simulink model "trabalhofinal_vR2012a"  (R2012a)
settings: Solver=FixedStepDiscrete  StartTime=0.0  StopTime=0.5  FixedStep=0.1e-6  MaxStep=50e-6
undefined symbols (not defined in the file): DiscIntNeverNeededParam, Ipac0, Vpac0
libraries: powerlib x36, simulink x19, fuzblock x7, powerlib_extras x2, powerlib_meascontrol x2
(part 2 of 3)

== system trabalhofinal_vR2012a/PV array PI/Compensador tensão ==
  Vdc* : Inport
  Vdc : Inport  Port=2
  Bus Creator : BusCreator  Inputs=3
  Constant1 : Constant  Value=Igq_e
  Cv(s) : simulink/Continuous/PID Controller  Controller=PI  TimeDomain=Discrete-time  SampleTime=-1  IntegratorMethod=Trapezoidal  FilterMethod=Forward Euler  Form=Parallel  UseFilter=on  ControllerParametersSource=internal  P=GSC_Cv_kp  I=GSC_Cv_ki  D=0  N=100  InitialConditionSource=external  InitialConditionForIntegrator=0  InitialConditionForFilter=0  ExternalReset=none  LimitOutput=off  UpperSaturationLimit=inf  LowerSaturationLimit=-inf  LinearizeAsGain=on  AntiWindupMode=none  Kb=1  TrackingMode=off  Kt=1  PParamMin=[]  PParamMax=[]  IParamMin=[]  IParamMax=[]  DParamMin=[]  DParamMax=[]  NParamMin=[]  NParamMax=[]  KbParamMin=[]  KbParamMax=[]  KtParamMin=[]  KtParamMax=[]  POutMin=[]  POutMax=[]  IOutMin=[]  IOutMax=[]  DOutMin=[]  DOutMax=[]  NOutMin=[]  NOutMax=[]  KbOutMin=[]  KbOutMax=[]  KtOutMin=[]  KtOutMax=[]  IntegratorOutMin=[]  IntegratorOutMax=[]  FilterOutMin=[]  FilterOutMax=[]  SumOutMin=[]  SumOutMax=[]  SumI1OutMin=[]  SumI1OutMax=[]  SumI2OutMin=[]  SumI2OutMax=[]  SumI3OutMin=[]  SumI3OutMax=[]  SumDOutMin=[]  SumDOutMax=[]  SaturationOutMin=[]  SaturationOutMax=[]  IntegratorContinuousStateAttributes=''  IntegratorStateMustResolveToSignalObject=off  IntegratorRTWStateStorageClass=Auto  FilterContinuousStateAttributes=''  FilterStateMustResolveToSignalObject=off  FilterRTWStateStorageClass=Auto  DifferentiatorICPrevScaledInput=0  DifferentiatorOutMin=[]  DifferentiatorOutMax=[]
  Gain : Gain  Gain=-1
  Scope5 : Scope  NumInputPorts=3
      settings: TimeRange=auto  MaxDataPoints=5000  SaveToWorkspace=off  SaveName=ScopeData2  YMin=2994.84204~2000.00000~589.79398  YMax=3046.42904~4000.00000~1186.78199  SampleTime=-1
  Sum1 : Sum  Inputs=|+-
  igq* : Outport
  DadosCtrlTensao : Outport  Port=2
  wires:
  Constant1/1 -> Cv(s)/2
  Vdc*/1 -> [vdc_ref], Sum1/1  "Vdc*"
  Vdc/1 -> [vdc], Sum1/2  "Vdc"
  Sum1/1 -> Gain/1
  [vdc] -> Scope5/1, Bus Creator/1  "vdc_V"
  [vdc_ref] -> Scope5/2, Bus Creator/2  "vdc_ref_V"
  [iqg_ref] -> Scope5/3, Bus Creator/3  "iqg_ref_A"
  Bus Creator/1 -> DadosCtrlTensao/1
  Gain/1 -> Cv(s)/1
  Cv(s)/1 -> [iqg_ref], igq*/1  "igq*"

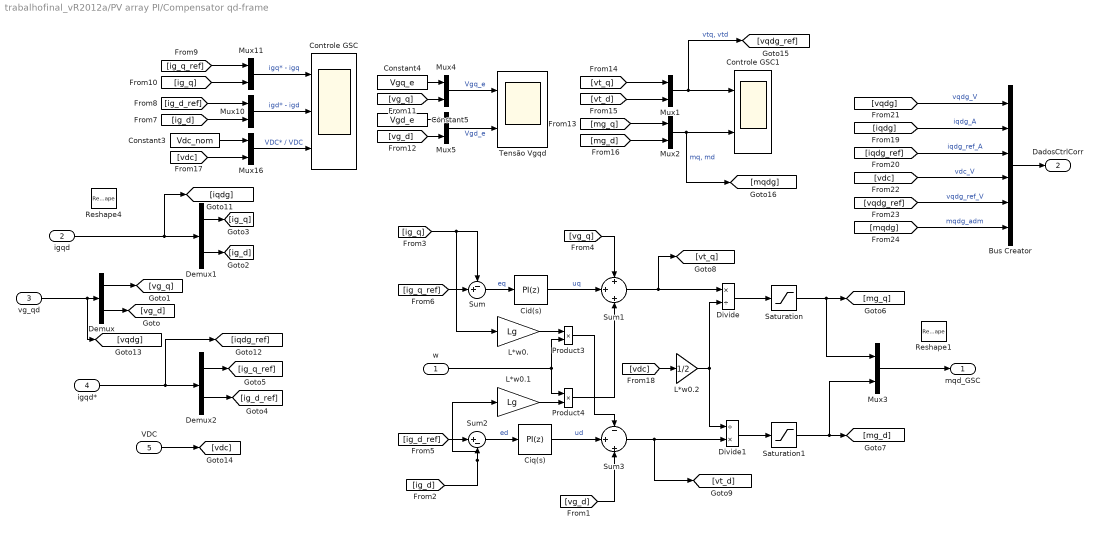
== system trabalhofinal_vR2012a/PV array PI/Compensator qd-frame ==
  w : Inport
  igqd : Inport  Port=2
  vg_qd : Inport  Port=3
  igqd* : Inport  Port=4
  VDC : Inport  Port=5
  Bus Creator : BusCreator  Inputs=6
  Cid(s) : simulink/Continuous/PID Controller  Controller=PI  TimeDomain=Discrete-time  SampleTime=-1  IntegratorMethod=Trapezoidal  FilterMethod=Forward Euler  Form=Parallel  UseFilter=on  ControllerParametersSource=internal  P=GSC_Ci_kp  I=GSC_Ci_ki  D=0  N=100  InitialConditionSource=internal  InitialConditionForIntegrator=GSC_Uq_e  InitialConditionForFilter=0  ExternalReset=none  LimitOutput=off  UpperSaturationLimit=inf  LowerSaturationLimit=-inf  LinearizeAsGain=on  AntiWindupMode=none  Kb=1  TrackingMode=off  Kt=1  PParamMin=[]  PParamMax=[]  IParamMin=[]  IParamMax=[]  DParamMin=[]  DParamMax=[]  NParamMin=[]  NParamMax=[]  KbParamMin=[]  KbParamMax=[]  KtParamMin=[]  KtParamMax=[]  POutMin=[]  POutMax=[]  IOutMin=[]  IOutMax=[]  DOutMin=[]  DOutMax=[]  NOutMin=[]  NOutMax=[]  KbOutMin=[]  KbOutMax=[]  KtOutMin=[]  KtOutMax=[]  IntegratorOutMin=[]  IntegratorOutMax=[]  FilterOutMin=[]  FilterOutMax=[]  SumOutMin=[]  SumOutMax=[]  SumI1OutMin=[]  SumI1OutMax=[]  SumI2OutMin=[]  SumI2OutMax=[]  SumI3OutMin=[]  SumI3OutMax=[]  SumDOutMin=[]  SumDOutMax=[]  SaturationOutMin=[]  SaturationOutMax=[]  IntegratorContinuousStateAttributes=''  IntegratorStateMustResolveToSignalObject=off  IntegratorRTWStateStorageClass=Auto  FilterContinuousStateAttributes=''  FilterStateMustResolveToSignalObject=off  FilterRTWStateStorageClass=Auto  DifferentiatorICPrevScaledInput=0  DifferentiatorOutMin=[]  DifferentiatorOutMax=[]
  Ciq(s) : simulink/Continuous/PID Controller  Controller=PI  TimeDomain=Discrete-time  SampleTime=-1  IntegratorMethod=Trapezoidal  FilterMethod=Forward Euler  Form=Parallel  UseFilter=on  ControllerParametersSource=internal  P=GSC_Ci_kp  I=GSC_Ci_ki  D=0  N=100  InitialConditionSource=internal  InitialConditionForIntegrator=GSC_Ud_e  InitialConditionForFilter=0  ExternalReset=none  LimitOutput=off  UpperSaturationLimit=inf  LowerSaturationLimit=-inf  LinearizeAsGain=on  AntiWindupMode=none  Kb=1  TrackingMode=off  Kt=1  PParamMin=[]  PParamMax=[]  IParamMin=[]  IParamMax=[]  DParamMin=[]  DParamMax=[]  NParamMin=[]  NParamMax=[]  KbParamMin=[]  KbParamMax=[]  KtParamMin=[]  KtParamMax=[]  POutMin=[]  POutMax=[]  IOutMin=[]  IOutMax=[]  DOutMin=[]  DOutMax=[]  NOutMin=[]  NOutMax=[]  KbOutMin=[]  KbOutMax=[]  KtOutMin=[]  KtOutMax=[]  IntegratorOutMin=[]  IntegratorOutMax=[]  FilterOutMin=[]  FilterOutMax=[]  SumOutMin=[]  SumOutMax=[]  SumI1OutMin=[]  SumI1OutMax=[]  SumI2OutMin=[]  SumI2OutMax=[]  SumI3OutMin=[]  SumI3OutMax=[]  SumDOutMin=[]  SumDOutMax=[]  SaturationOutMin=[]  SaturationOutMax=[]  IntegratorContinuousStateAttributes=''  IntegratorStateMustResolveToSignalObject=off  IntegratorRTWStateStorageClass=Auto  FilterContinuousStateAttributes=''  FilterStateMustResolveToSignalObject=off  FilterRTWStateStorageClass=Auto  DifferentiatorICPrevScaledInput=0  DifferentiatorOutMin=[]  DifferentiatorOutMax=[]
  Constant3 : Constant  Value=Vdc_nom
  Constant4 : Constant  Value=Vgq_e
  Constant5 : Constant  Value=Vgd_e
  Controle GSC : Scope  NumInputPorts=3
      settings: TimeRange=0.1  MaxDataPoints=5000  SaveToWorkspace=off  SaveName=ScopeData3  YMin=-63.17117~-5.51729~796.71882  YMax=425.59411~20.68997~829.53063  SampleTime=-1
  Controle GSC1 : Scope  NumInputPorts=2
      settings: TimeRange=auto  MaxDataPoints=5000  SaveToWorkspace=off  SaveName=ScopeData4  YMin=-135.91868~-0.45232  YMax=350.40738~1.16137  SampleTime=-1
  Demux : Demux  Outputs=2
  Demux1 : Demux  Outputs=2
  Demux2 : Demux  Outputs=2
  Divide : Product  Inputs=*/
  Divide1 : Product  Inputs=/*
  L*w0. : Gain  Gain=Lg
  L*w0.1 : Gain  Gain=Lg
  L*w0.2 : Gain  Gain=1/2
  Mux{1..5,10..11,16} (8 alike) : Mux  Inputs=2
  Product3 : Product
  Product4 : Product
  Reshape1 : Reshape  OutputDimensionality=Customize  OutputDimensions=[2,1]
  Reshape4 : Reshape  OutputDimensionality=Customize  OutputDimensions=[2,1]
  Saturation : Saturate  UpperLimit=1  LowerLimit=-1
  Saturation1 : Saturate  UpperLimit=1  LowerLimit=-1
  Sum : Sum  Inputs=-+|
  Sum1 : Sum  Inputs=+|+|+
  Sum2 : Sum  Inputs=|+-
  Sum3 : Sum  Inputs=-|+|+
  Tensão Vgqd : Scope  NumInputPorts=2
      settings: TimeRange=auto  MaxDataPoints=5000  SaveToWorkspace=off  SaveName=ScopeData36  YMin=148.66619~-14.34464  YMax=209.64626~12.14165  SampleTime=-1
  mqd_GSC : Outport
  DadosCtrlCorr : Outport  Port=2
  wires:
  Demux/2 -> [vg_d]
  Demux/1 -> [vg_q]
  Demux1/2 -> [ig_d]
  Demux1/1 -> [ig_q]
  L*w0.2/1 -> Divide/2, Divide1/1
  [mg_q] -> Mux2/1
  [mg_d] -> Mux2/2
  [vt_q] -> Mux1/1
  [vt_d] -> Mux1/2
  Mux2/1 -> [mqdg], Controle GSC1/2  "mq, md"
  Mux1/1 -> [vqdg_ref], Controle GSC1/1  "vtq, vtd"
  [ig_q] -> Mux11/2
  [ig_q_ref] -> Mux11/1
  [ig_d] -> Mux10/2
  [ig_d_ref] -> Mux10/1
  Mux11/1 -> Controle GSC/1  "igq* - igq"
  Mux10/1 -> Controle GSC/2  "igd* - igd"
  Divide/1 -> Saturation/1
  L*w0.1/1 -> Product4/2
  [ig_q_ref] -> Sum/2
  igqd*/1 -> Demux2/1, [iqdg_ref]
  VDC/1 -> [vdc]
  Sum/1 -> Cid(s)/1  "eq"
  [ig_d] -> L*w0.1/1, Sum2/2
  Sum1/1 -> Divide/1, [vt_q]
  Cid(s)/1 -> Sum1/2  "uq"
  Ciq(s)/1 -> Sum3/2  "ud"
  Sum2/1 -> Ciq(s)/1  "ed"
  Sum3/1 -> Divide1/2, [vt_d]
  L*w0./1 -> Product3/1
  [ig_d_ref] -> Sum2/1
  Mux16/1 -> Controle GSC/3  "VDC* / VDC"
  Constant3/1 -> Mux16/1
  [vdc] -> Mux16/2
  Demux2/1 -> [ig_q_ref]
  Demux2/2 -> [ig_d_ref]
  [vdc] -> L*w0.2/1
  Constant4/1 -> Mux4/1
  [vg_q] -> Mux4/2
  Constant5/1 -> Mux5/1
  [vg_d] -> Mux5/2
  Mux4/1 -> Tensão Vgqd/1  "Vgq_e"
  Mux5/1 -> Tensão Vgqd/2  "Vgd_e"
  Saturation/1 -> Mux3/1, [mg_q]
  Divide1/1 -> Saturation1/1
  Saturation1/1 -> Mux3/2, [mg_d]
  [ig_q] -> Sum/1, L*w0./1
  igqd/1 -> [iqdg], Demux1/1
  vg_qd/1 -> [vqdg], Demux/1
  Mux3/1 -> mqd_GSC/1
  [vqdg] -> Bus Creator/1  "vqdg_V"
  [iqdg] -> Bus Creator/2  "iqdg_A"
  [iqdg_ref] -> Bus Creator/3  "iqdg_ref_A"
  Bus Creator/1 -> DadosCtrlCorr/1
  [vdc] -> Bus Creator/4  "vdc_V"
  [vqdg_ref] -> Bus Creator/5  "vqdg_ref_V"
  [mqdg] -> Bus Creator/6  "mqdg_adm"
  [vg_q] -> Sum1/1
  [vg_d] -> Sum3/3
  Product3/1 -> Sum3/1
  Product4/1 -> Sum1/3
  w/1 -> Product3/2, Product4/1

== system trabalhofinal_vR2012a/PV array PI/DSOGI1 ==
  note: Fasor = (Fq-jFd)/sqrt(2)
  angV : Inport
  V : Inport  Port=2
  I : Inport  Port=3
  Calcula Impedância2 : Subsystem
  Complex to Magnitude-Angle : ComplexToMagnitudeAngle  Output=Angle
  Complex to Magnitude-Angle1 : ComplexToMagnitudeAngle
  Fasor_Krause : Subsystem
  Fasor_Krause1 : Subsystem
  Magnitude-Angle to Complex : MagnitudeAngleToComplex
  Sum : Sum  Inputs=|++
  Terminator : Terminator
  I_fasor : Outport
  wires:
  Magnitude-Angle to Complex/1 -> I_fasor/1
  Complex to Magnitude-Angle1/2 -> Sum/1
  Complex to Magnitude-Angle1/1 -> Magnitude-Angle to Complex/1
  Complex to Magnitude-Angle/1 -> Terminator/1
  V/1 -> Calcula Impedância2/1(Vinf_abc)
  I/1 -> Calcula Impedância2/2(I_abc)
  Calcula Impedância2/1(Vinf_q) -> Fasor_Krause/1(Fq)
  Calcula Impedância2/2(Vinf_d) -> Fasor_Krause/2(Fd)
  Fasor_Krause/1(Fasor) -> Complex to Magnitude-Angle/1
  Calcula Impedância2/3(Ipac_q) -> Fasor_Krause1/1(Fq)
  Calcula Impedância2/4(Ipac_d) -> Fasor_Krause1/2(Fd)
  Fasor_Krause1/1(Fasor) -> Complex to Magnitude-Angle1/1
  Sum/1 -> Magnitude-Angle to Complex/2
  angV/1 -> Sum/2

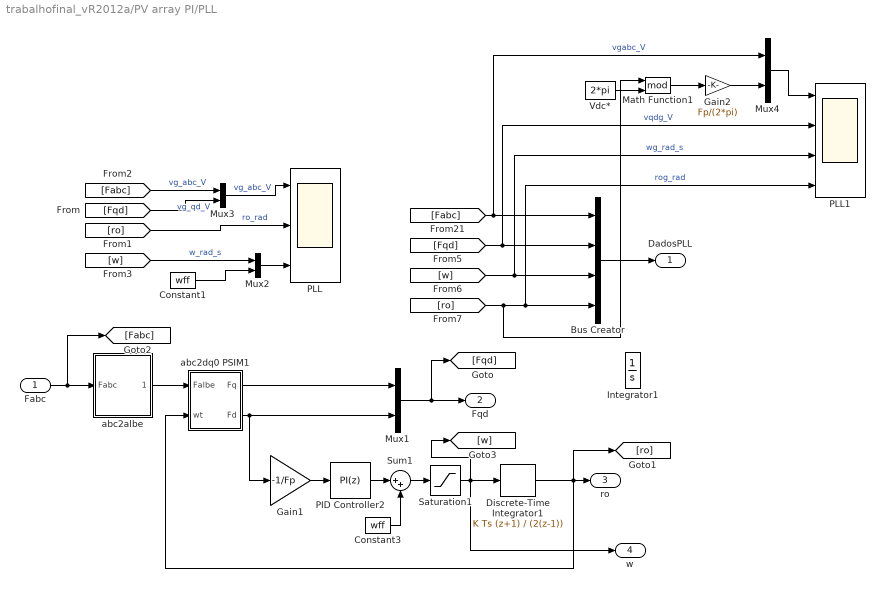
== system trabalhofinal_vR2012a/PV array PI/PLL ==
  Fabc : Inport
  Bus Creator : BusCreator  Inputs=4
  Constant1 : Constant  Value=wff
  Constant3 : Constant  Value=wff
  Discrete-Time Integrator1 : DiscreteIntegrator  IntegratorMethod=Integration: Trapezoidal  InitialCondition=ro0  InitialConditionMode=State only (most efficient)  SampleTime=-1  ICPrevOutput=DiscIntNeverNeededParam  ICPrevScaledInput=DiscIntNeverNeededParam
  Gain1 : Gain  Gain=-1/Fp
  Gain2 : Gain  Gain=Fp/(2*pi)
  Integrator1 : Integrator  InitialCondition=ro0  UpperSaturationLimit=2*pi  LowerSaturationLimit=0
  Math Function1 : Math  Operator=mod  SaturateOnIntegerOverflow=on
  Mux{1..4} (4 alike) : Mux  Inputs=2
  PID Controller2 : simulink/Continuous/PID Controller  Controller=PI  TimeDomain=Discrete-time  SampleTime=-1  IntegratorMethod=Trapezoidal  FilterMethod=Forward Euler  Form=Parallel  UseFilter=on  ControllerParametersSource=internal  P=kp  I=ki  D=1  N=100  InitialConditionSource=internal  InitialConditionForIntegrator=dw0  InitialConditionForFilter=0  ExternalReset=none  LimitOutput=off  UpperSaturationLimit=inf  LowerSaturationLimit=-inf  LinearizeAsGain=on  AntiWindupMode=none  Kb=1  TrackingMode=off  Kt=1  PParamMin=[]  PParamMax=[]  IParamMin=[]  IParamMax=[]  DParamMin=[]  DParamMax=[]  NParamMin=[]  NParamMax=[]  KbParamMin=[]  KbParamMax=[]  KtParamMin=[]  KtParamMax=[]  POutMin=[]  POutMax=[]  IOutMin=[]  IOutMax=[]  DOutMin=[]  DOutMax=[]  NOutMin=[]  NOutMax=[]  KbOutMin=[]  KbOutMax=[]  KtOutMin=[]  KtOutMax=[]  IntegratorOutMin=[]  IntegratorOutMax=[]  FilterOutMin=[]  FilterOutMax=[]  SumOutMin=[]  SumOutMax=[]  SumI1OutMin=[]  SumI1OutMax=[]  SumI2OutMin=[]  SumI2OutMax=[]  SumI3OutMin=[]  SumI3OutMax=[]  SumDOutMin=[]  SumDOutMax=[]  SaturationOutMin=[]  SaturationOutMax=[]  IntegratorContinuousStateAttributes=''  IntegratorStateMustResolveToSignalObject=off  IntegratorRTWStateStorageClass=Auto  FilterContinuousStateAttributes=''  FilterStateMustResolveToSignalObject=off  FilterRTWStateStorageClass=Auto  DifferentiatorICPrevScaledInput=0  DifferentiatorOutMin=[]  DifferentiatorOutMax=[]
  PLL : Scope  NumInputPorts=3
      settings: TimeRange=auto  MaxDataPoints=5000  SaveToWorkspace=off  SaveName=ScopeData  YMin=-224.53656~-6.47953~126.78086  YMax=224.53656~42.60785~2394.62118  SampleTime=-1
  PLL1 : Scope  NumInputPorts=4
      settings: TimeRange=auto  MaxDataPoints=5000  SaveToWorkspace=off  SaveName=ScopeData2  YMin=-449.07312~-45.53757~341.99428~-25.11328  YMax=449.07312~404.23584~381.19293~210.48455  SampleTime=-1
  Saturation1 : Saturate  UpperLimit=10*wff  LowerLimit=-0.1*wff
  Sum1 : Sum  Inputs=|++
  Vdc* : Constant  Value=2*pi  SampleTime=-1
  abc2albe : Subsystem
  abc2dq0 PSIM1 : Subsystem
  DadosPLL : Outport
  Fqd : Outport  Port=2
  ro : Outport  Port=3
  w : Outport  Port=4
  wires:
  abc2albe/1(Falbe) -> abc2dq0 PSIM1/1(Falbe)
  abc2dq0 PSIM1/2(Fd) -> Gain1/1, Mux1/2
  Constant3/1 -> Sum1/2
  abc2dq0 PSIM1/1(Fq) -> Mux1/1
  Sum1/1 -> Saturation1/1
  Gain1/1 -> PID Controller2/1
  PID Controller2/1 -> Sum1/1
  Mux3/1 -> PLL/1  "vg_abc_V"
  Fabc/1 -> abc2albe/1(Fabc), [Fabc]
  [ro] -> PLL/2  "ro_rad"
  [Fqd] -> Mux3/2  "vg_qd_V"
  Mux1/1 -> Fqd/1, [Fqd]
  [w] -> Mux2/1  "w_rad_s"
  Mux2/1 -> PLL/3
  Constant1/1 -> Mux2/2
  [Fabc] -> Mux4/1, Bus Creator/1  "vgabc_V"
  [Fqd] -> PLL1/2, Bus Creator/2  "vqdg_V"
  [w] -> PLL1/3, Bus Creator/3  "wg_rad_s"
  Bus Creator/1 -> DadosPLL/1
  [ro] -> Math Function1/1, PLL1/4, Bus Creator/4  "rog_rad"
  [Fabc] -> Mux3/1  "vg_abc_V"
  Saturation1/1 -> w/1, Discrete-Time Integrator1/1, [w]
  Discrete-Time Integrator1/1 -> [ro], abc2dq0 PSIM1/2(wt), ro/1
  Vdc*/1 -> Math Function1/2
  Math Function1/1 -> Gain2/1
  Mux4/1 -> PLL1/1
  Gain2/1 -> Mux4/2

== system trabalhofinal_vR2012a/PV array PI/PWM ==
  mabc : Inport
  PWM Generator1 : powerlib_extras/Control  Blocks/PWM Generator  GeneratorMode="3-arm  bridge (6 pulses)"  Fc=PWM_freq_grid  Internal=off  mIndex=0.4  Freq=60  Phase=0
  Unit Delay4 : UnitDelay  SampleTime=-1
  Pulses : Outport
  wires:
  PWM Generator1/1 -> Pulses/1
  mabc/1 -> PWM Generator1/1

== system trabalhofinal_vR2012a/PV array PI/Subsystem ==
  Current Measurement : powerlib/Measurements/Current Measurement  PhasorSimulation=off  OutputType=Complex  PSBequivalent=0
  vbn : powerlib/Measurements/Voltage Measurement  PhasorSimulation=off  OutputType=Complex  PSBequivalent=0
  A : PMIOPort  Port=1  Side=Left
  a : PMIOPort  Port=2  Side=Right
  B : PMIOPort  Port=3  Side=Left
  Vdc : Outport
  Idc : Outport  Port=2
  wires:
  Current Measurement/1 -> Idc/1
  vbn/1 -> Vdc/1
  connections:
  Current Measurement/LConn1 -- a/RConn1
  vbn/LConn2 -- B/RConn1
  vbn/LConn1 -- A/RConn1 -- Current Measurement/RConn1

== system trabalhofinal_vR2012a/PV array PI/abc2dq0 PSIM1 ==
  Fabc : Inport
  wt : Inport  Port=2
  Mux1 : Mux  Inputs=2
  abc2albe : Subsystem
  abc2dq0 PSIM1 : Subsystem
  Fqd : Outport
  wires:
  abc2albe/1(Falbe) -> abc2dq0 PSIM1/1(Falbe)
  abc2dq0 PSIM1/2(Fd) -> Mux1/2
  abc2dq0 PSIM1/1(Fq) -> Mux1/1
  Mux1/1 -> Fqd/1
  wt/1 -> abc2dq0 PSIM1/2(wt)
  Fabc/1 -> abc2albe/1(Fabc)

== system trabalhofinal_vR2012a/PV array PI/dq02abc PSIM ==
  Fqd : Inport
  wt : Inport  Port=2
  abc2dq0 PSIM : Subsystem
  albe2abc : Subsystem
  Fabc : Outport
  wires:
  albe2abc/1(Fabc) -> Fabc/1
  abc2dq0 PSIM/1(Falbe) -> albe2abc/1(Falbe)
  wt/1 -> abc2dq0 PSIM/2(wt)
  Fqd/1 -> abc2dq0 PSIM/1(Fqd)

== system trabalhofinal_vR2012a/PV array Fuzzy/Compensador tensão/F1 ==
  E : Inport
  Fuzzy Logic Controller1 : fuzblock/Fuzzy Logic  Controller  fis=fuzzyControl
  Gain9 : Gain  Gain=GY
  Mux6 : Mux  Inputs=2
  Rate Transition1 : RateTransition  OutPortSampleTime=Ts_fuzzy
  Rate Transition2 : RateTransition
  Saturation2 : Saturate  UpperLimit=1  LowerLimit=-1
  Scope5 : Scope  NumInputPorts=3
      settings: TimeRange=auto  MaxDataPoints=5000  SaveToWorkspace=off  YMin=-1.25~-0.09079~-1.05  YMax=1.25~0.07544~1.05  SampleTime=-1
  Subsystem1 : Subsystem
  u : Outport
  wires:
  Rate Transition1/1 -> Subsystem1/1(E)
  Saturation2/1 -> Gain9/1
  Subsystem1/1(E.) -> Mux6/1, Scope5/1  "E"
  Mux6/1 -> Fuzzy Logic Controller1/1
  Subsystem1/2(CE) -> Mux6/2, Scope5/2  "CE"
  Fuzzy Logic Controller1/1 -> Scope5/3, Saturation2/1  "u"
  Gain9/1 -> Rate Transition2/1
  E/1 -> Rate Transition1/1
  Rate Transition2/1 -> u/1

== system trabalhofinal_vR2012a/PV array Fuzzy/Compensador tensão/F2 ==
  E : Inport
  Fuzzy Logic Controller1 : fuzblock/Fuzzy Logic  Controller  fis=fuzzyControl
  Gain9 : Gain  Gain=GY
  Mux6 : Mux  Inputs=2
  Rate Transition1 : RateTransition  OutPortSampleTime=Ts_fuzzy
  Rate Transition2 : RateTransition
  Saturation2 : Saturate  UpperLimit=1  LowerLimit=-1
  Scope5 : Scope  NumInputPorts=3
      settings: TimeRange=auto  MaxDataPoints=5000  SaveToWorkspace=off  YMin=-1.25~-0.66794~-1.05  YMax=1.25~1.18533~1.05  SampleTime=-1
  Subsystem1 : Subsystem
  u : Outport
  wires:
  Rate Transition2/1 -> u/1
  E/1 -> Rate Transition1/1
  Gain9/1 -> Rate Transition2/1
  Fuzzy Logic Controller1/1 -> Saturation2/1, Scope5/3  "u"
  Subsystem1/2(CE) -> Scope5/2, Mux6/2  "CE"
  Mux6/1 -> Fuzzy Logic Controller1/1
  Subsystem1/1(E.) -> Scope5/1, Mux6/1  "E"
  Saturation2/1 -> Gain9/1
  Rate Transition1/1 -> Subsystem1/1(E)

== system trabalhofinal_vR2012a/PV array Fuzzy/Compensador tensão/F3 ==
  E : Inport
  Fuzzy Logic Controller1 : fuzblock/Fuzzy Logic  Controller  fis=fuzzyControl
  Gain9 : Gain  Gain=GY
  Mux6 : Mux  Inputs=2
  Rate Transition1 : RateTransition  OutPortSampleTime=Ts_fuzzy
  Rate Transition2 : RateTransition
  Saturation2 : Saturate  UpperLimit=1  LowerLimit=-1
  Scope5 : Scope  NumInputPorts=3
      settings: TimeRange=auto  MaxDataPoints=5000  SaveToWorkspace=off  YMin=-0.08604~-0.00307~-0.07636  YMax=0.77447~0.01457~0.68814  SampleTime=-1
  Subsystem1 : Subsystem
  u : Outport
  wires:
  Rate Transition1/1 -> Subsystem1/1(E)
  Saturation2/1 -> Gain9/1
  Subsystem1/1(E.) -> Mux6/1, Scope5/1  "E"
  Mux6/1 -> Fuzzy Logic Controller1/1
  Subsystem1/2(CE) -> Mux6/2, Scope5/2  "CE"
  Fuzzy Logic Controller1/1 -> Scope5/3, Saturation2/1  "u"
  Gain9/1 -> Rate Transition2/1
  E/1 -> Rate Transition1/1
  Rate Transition2/1 -> u/1

== system trabalhofinal_vR2012a/PV array Fuzzy/Compensador tensão/F4 ==
  E : Inport
  Fuzzy Logic Controller1 : fuzblock/Fuzzy Logic  Controller  fis=fuzzyControl
  Gain9 : Gain  Gain=GY
  Mux6 : Mux  Inputs=2
  Rate Transition1 : RateTransition  OutPortSampleTime=Ts_fuzzy
  Rate Transition2 : RateTransition
  Saturation2 : Saturate  UpperLimit=1  LowerLimit=-1
  Scope5 : Scope  NumInputPorts=3
      settings: TimeRange=auto  MaxDataPoints=5000  SaveToWorkspace=off  YMin=-0.0901~-0.00492~-0.07806  YMax=0.81164~0.01477~0.70508  SampleTime=-1
  Subsystem1 : Subsystem
  u : Outport
  wires:
  Rate Transition1/1 -> Subsystem1/1(E)
  Saturation2/1 -> Gain9/1
  Subsystem1/1(E.) -> Mux6/1, Scope5/1  "E"
  Mux6/1 -> Fuzzy Logic Controller1/1
  Subsystem1/2(CE) -> Mux6/2, Scope5/2  "CE"
  Fuzzy Logic Controller1/1 -> Scope5/3, Saturation2/1  "u"
  Gain9/1 -> Rate Transition2/1
  E/1 -> Rate Transition1/1
  Rate Transition2/1 -> u/1

== system trabalhofinal_vR2012a/PV array Fuzzy/Compensador tensão/Ganhos1 ==
  E : Inport
  Fuzzy Logic Controller1 : fuzblock/Fuzzy Logic  Controller  fis=fuzzyControl
  Gain9 : Gain  Gain=GY
  Mux6 : Mux  Inputs=2
  Rate Transition1 : RateTransition  OutPortSampleTime=Ts_fuzzy
  Saturation2 : Saturate  UpperLimit=1  LowerLimit=-1
  Scope5 : Scope  NumInputPorts=3
      settings: TimeRange=auto  MaxDataPoints=5000  SaveToWorkspace=off  YMin=-0.36602~-1.25~-1.04912  YMax=0.83247~1.25~1.04987  SampleTime=-1
  Subsystem1 : Subsystem
  u : Outport
  wires:
  Gain9/1 -> u/1
  E/1 -> Rate Transition1/1
  Fuzzy Logic Controller1/1 -> Saturation2/1, Scope5/3  "u"
  Subsystem1/2(CE) -> Scope5/2, Mux6/2  "CE"
  Mux6/1 -> Fuzzy Logic Controller1/1
  Subsystem1/1(E.) -> Scope5/1, Mux6/1  "E"
  Saturation2/1 -> Gain9/1
  Rate Transition1/1 -> Subsystem1/1(E)

== system trabalhofinal_vR2012a/PV array Fuzzy/Compensador tensão/Subsystem1 ==
  E : Inport
  Discrete Derivative1 : simulink/Discrete/Discrete Derivative  gainval=1  ICPrevScaledInput=0.0  OutMin=[]  OutMax=[]  OutDataType=fixdt(1, 16)  OutScaling=2^-10  DoSatur=off
  E. : Outport
  CE : Outport  Port=2
  wires:
  E/1 -> E./1, Discrete Derivative1/1
  Discrete Derivative1/1 -> CE/1  "CE"

== system trabalhofinal_vR2012a/PV array Fuzzy/Compensador tensão/razoável ==
  E : Inport
  Fuzzy Logic Controller1 : fuzblock/Fuzzy Logic  Controller  fis=teste03
  Gain9 : Gain  Gain=GY
  Mux6 : Mux  Inputs=2
  Rate Transition1 : RateTransition  OutPortSampleTime=0.0001
  Rate Transition2 : RateTransition
  Saturation2 : Saturate  UpperLimit=1  LowerLimit=-1
  Scope5 : Scope  NumInputPorts=3
      settings: TimeRange=auto  MaxDataPoints=5000  SaveToWorkspace=off  YMin=-0.03774~-0.02191~-0.05244  YMax=0.33999~0.07353~0.47629  SampleTime=-1
  Subsystem1 : Subsystem
  u : Outport
  wires:
  Saturation2/1 -> Gain9/1
  Subsystem1/1(E.) -> Mux6/1, Scope5/1  "E"
  Mux6/1 -> Fuzzy Logic Controller1/1
  Subsystem1/2(CE) -> Mux6/2, Scope5/2  "CE"
  Fuzzy Logic Controller1/1 -> Scope5/3, Saturation2/1  "u"
  Gain9/1 -> Rate Transition2/1
  E/1 -> Rate Transition1/1
  Rate Transition1/1 -> Subsystem1/1(E)
  Rate Transition2/1 -> u/1

== system trabalhofinal_vR2012a/PV array Fuzzy/Compensator qd-frame/FuzzyControl_q3 ==
  E : Inport
  Fuzzy Logic Controller1 : fuzblock/Fuzzy Logic  Controller  fis=teste03
  Gain9 : Gain  Gain=GY
  Mux6 : Mux  Inputs=2
  Rate Transition1 : RateTransition  OutPortSampleTime=0.0001
  Rate Transition2 : RateTransition
  Saturation2 : Saturate  UpperLimit=1  LowerLimit=-1
  Scope5 : Scope  NumInputPorts=3
      settings: TimeRange=auto  MaxDataPoints=5000  SaveToWorkspace=off  YMin=-0.34895~-1.25~-1.04994  YMax=1.14988~1.25~1.04999  SampleTime=-1
  Subsystem1 : Subsystem
  u : Outport
  wires:
  Rate Transition2/1 -> u/1
  Rate Transition1/1 -> Subsystem1/1(E)
  E/1 -> Rate Transition1/1
  Gain9/1 -> Rate Transition2/1
  Fuzzy Logic Controller1/1 -> Saturation2/1, Scope5/3  "u"
  Subsystem1/2(CE) -> Scope5/2, Mux6/2  "CE"
  Mux6/1 -> Fuzzy Logic Controller1/1
  Subsystem1/1(E.) -> Scope5/1, Mux6/1  "E"
  Saturation2/1 -> Gain9/1

== system trabalhofinal_vR2012a/PV array Fuzzy/Compensator qd-frame/Subsystem2 ==
  E : Inport
  Discrete Derivative1 : simulink/Discrete/Discrete Derivative  gainval=1  ICPrevScaledInput=0.0  OutMin=[]  OutMax=[]  OutDataType=fixdt(1, 16)  OutScaling=2^-10  DoSatur=off
  Gain8 : Gain
  Gain9 : Gain
  Saturation2 : Saturate  UpperLimit=inf  LowerLimit=-inf
  E. : Outport
  CE : Outport  Port=2
  wires:
  Gain9/1 -> E./1
  Saturation2/1 -> CE/1
  E/1 -> Discrete Derivative1/1, Gain9/1
  Discrete Derivative1/1 -> Gain8/1  "CE"
  Gain8/1 -> Saturation2/1

== system trabalhofinal_vR2012a/PV array Fuzzy/DSOGI1/Calcula Impedância2 ==
  Vinf_abc : Inport
  I_abc : Inport  Port=2
  Constant2 : Constant  Value=wB  SampleTime=0
  DSOGI (Corrente) : Subsystem
  DSOGI (Tensão) : Subsystem
  Demux : Demux  Outputs=2
  Demux1 : Demux  Outputs=2
  Gain : Gain
  PLL : Subsystem
  PLL1 : Scope  NumInputPorts=2
      settings: TimeRange=auto  MaxDataPoints=5000  SaveToWorkspace=off  SaveName=ScopeData5  YMin=-1.5~-0.25  YMax=1.5~1.5  SampleTime=-1
  PLL2 : Scope  NumInputPorts=2
      settings: TimeRange=auto  MaxDataPoints=5000  SaveToWorkspace=off  YMin=-1.5~-0.25  YMax=1.5~1.5  SampleTime=-1
  Sum1 : Sum  Inputs=+-|
  Terminator6 : Terminator
  Terminator7 : Terminator
  abc2albe : Subsystem
  abc2albe1 : Subsystem
  abc2dq0 PSIM : Subsystem
  Vinf_q : Outport
  Vinf_d : Outport  Port=2
  Ipac_q : Outport  Port=3
  Ipac_d : Outport  Port=4
  wires:
  Gain/1 -> Sum1/2
  I_abc/1 -> abc2albe1/1(Fabc)
  PLL/3(ro) -> PLL/2(wt), abc2dq0 PSIM/2(wt)
  DSOGI (Corrente)/1(Falbe(+)) -> PLL1/1, abc2dq0 PSIM/1(Falbe)
  DSOGI (Corrente)/2(Falbe(-)) -> Terminator7/1
  abc2albe1/1(Falbe) -> DSOGI (Corrente)/2(Falbe)
  DSOGI (Tensão)/2(Falbe(-)) -> Terminator6/1
  Vinf_abc/1 -> abc2albe/1(Fabc)
  DSOGI (Tensão)/1(Falbe(+)) -> PLL/1(Falbe)
  abc2albe/1(Falbe) -> DSOGI (Tensão)/2(Falbe)
  PLL/1(Fqd) -> Demux/1, PLL2/1
  Demux1/2 -> Ipac_d/1
  Demux/2 -> Vinf_d/1
  Demux/1 -> Vinf_q/1
  abc2dq0 PSIM/1(Fqd) -> PLL1/2, Demux1/1
  Demux1/1 -> Ipac_q/1
  PLL/2(w) -> PLL2/2
  Constant2/1 -> DSOGI (Corrente)/1(w), DSOGI (Tensão)/1(w)

== system trabalhofinal_vR2012a/PV array Fuzzy/DSOGI1/Fasor_Krause ==
  Fq : Inport
  Fd : Inport  Port=2
  Gain12 : Gain  Gain=-1
  Gain7 : Gain  Gain=1/sqrt(2)
  Real-Imag to Complex1 : RealImagToComplex
  Fasor : Outport
  wires:
  Real-Imag to Complex1/1 -> Gain7/1
  Fq/1 -> Real-Imag to Complex1/1
  Gain12/1 -> Real-Imag to Complex1/2
  Fd/1 -> Gain12/1
  Gain7/1 -> Fasor/1

== system trabalhofinal_vR2012a/PV array Fuzzy/DSOGI1/Fasor_Krause1 ==
  Fq : Inport
  Fd : Inport  Port=2
  Gain12 : Gain  Gain=-1
  Gain7 : Gain  Gain=1/sqrt(2)
  Real-Imag to Complex1 : RealImagToComplex
  Fasor : Outport
  wires:
  Gain7/1 -> Fasor/1
  Fd/1 -> Gain12/1
  Gain12/1 -> Real-Imag to Complex1/2
  Fq/1 -> Real-Imag to Complex1/1
  Real-Imag to Complex1/1 -> Gain7/1

== system trabalhofinal_vR2012a/PV array Fuzzy/PLL/abc2albe ==
  Fabc : Inport
  Gain1 : Gain  Gain=2/3  SaturateOnIntegerOverflow=on  OutDataTypeStr=Inherit: Same as input  ParamDataTypeStr=Inherit: Same as input
  Gain3 : Gain  Gain="[ 1   -1/2   -1/2; 0   sqrt(3)/2   -sqrt(3)/2 ]"  Multiplication=Matrix(K*u) (u vector)  SaturateOnIntegerOverflow=on  OutDataTypeStr=Inherit: Same as input  ParamDataTypeStr=Inherit: Same as input
  Falbe : Outport
  wires:
  Gain1/1 -> Falbe/1
  Gain3/1 -> Gain1/1
  Fabc/1 -> Gain3/1

== system trabalhofinal_vR2012a/PV array Fuzzy/PLL/abc2dq0 PSIM1 ==
  Falbe : Inport
  wt : Inport  Port=2
  Fcn1 : Fcn  Expr=u(1)*cos(u(3))+u(2)*sin(u(3))
  Fcn2 : Fcn  Expr=u(1)*sin(u(3))-u(2)*cos(u(3))
  Mux : Mux  Inputs=2
  Fq : Outport
  Fd : Outport  Port=2
  wires:
  Mux/1 -> Fcn1/1, Fcn2/1
  wt/1 -> Mux/2
  Fcn2/1 -> Fd/1
  Fcn1/1 -> Fq/1
  Falbe/1 -> Mux/1

== system trabalhofinal_vR2012a/PV array Fuzzy/abc2dq0 PSIM1/abc2albe ==
  Fabc : Inport
  Gain1 : Gain  Gain=2/3  SaturateOnIntegerOverflow=on  OutDataTypeStr=Inherit: Same as input  ParamDataTypeStr=Inherit: Same as input
  Gain3 : Gain  Gain="[ 1   -1/2   -1/2; 0   sqrt(3)/2   -sqrt(3)/2 ]"  Multiplication=Matrix(K*u) (u vector)  SaturateOnIntegerOverflow=on  OutDataTypeStr=Inherit: Same as input  ParamDataTypeStr=Inherit: Same as input
  Falbe : Outport
  wires:
  Gain1/1 -> Falbe/1
  Gain3/1 -> Gain1/1
  Fabc/1 -> Gain3/1

== system trabalhofinal_vR2012a/PV array Fuzzy/abc2dq0 PSIM1/abc2dq0 PSIM1 ==
  Falbe : Inport
  wt : Inport  Port=2
  Fcn1 : Fcn  Expr=u(1)*cos(u(3))+u(2)*sin(u(3))
  Fcn2 : Fcn  Expr=u(1)*sin(u(3))-u(2)*cos(u(3))
  Mux : Mux  Inputs=2
  Fq : Outport
  Fd : Outport  Port=2
  wires:
  Mux/1 -> Fcn1/1, Fcn2/1
  wt/1 -> Mux/2
  Fcn2/1 -> Fd/1
  Fcn1/1 -> Fq/1
  Falbe/1 -> Mux/1

== system trabalhofinal_vR2012a/PV array Fuzzy/dq02abc PSIM/abc2dq0 PSIM ==
  Fqd : Inport
  wt : Inport  Port=2
  Fcn1 : Fcn  Expr=u(1)*cos(u(3))+u(2)*sin(u(3))
  Fcn2 : Fcn  Expr=u(1)*sin(u(3))-u(2)*cos(u(3))
  Mux : Mux  Inputs=2
  Mux1 : Mux  Inputs=2
  Falbe : Outport
  wires:
  Mux1/1 -> Falbe/1
  Mux/1 -> Fcn1/1, Fcn2/1
  wt/1 -> Mux/2
  Fcn2/1 -> Mux1/2
  Fcn1/1 -> Mux1/1
  Fqd/1 -> Mux/1

== system trabalhofinal_vR2012a/PV array Fuzzy/dq02abc PSIM/albe2abc ==
  Falbe : Inport
  Gain3 : Gain  Gain="[ 1   0; -1/2  sqrt(3)/2; -1/2  -sqrt(3)/2]"  Multiplication=Matrix(K*u) (u vector)  SaturateOnIntegerOverflow=on  OutDataTypeStr=Inherit: Same as input  ParamDataTypeStr=Inherit: Same as input
  Fabc : Outport
  wires:
  Gain3/1 -> Fabc/1
  Falbe/1 -> Gain3/1

== system trabalhofinal_vR2012a/PV array PI/DSOGI1/Calcula Impedância2 ==
  Vinf_abc : Inport
  I_abc : Inport  Port=2
  Constant2 : Constant  Value=wB  SampleTime=0
  DSOGI (Corrente) : Subsystem
  DSOGI (Tensão) : Subsystem
  Demux : Demux  Outputs=2
  Demux1 : Demux  Outputs=2
  Gain : Gain
  PLL : Subsystem
  PLL1 : Scope  NumInputPorts=2
      settings: TimeRange=auto  MaxDataPoints=5000  SaveToWorkspace=off  SaveName=ScopeData5  YMin=-1.5~-0.25  YMax=1.5~1.5  SampleTime=-1
  PLL2 : Scope  NumInputPorts=2
      settings: TimeRange=auto  MaxDataPoints=5000  SaveToWorkspace=off  YMin=-1.5~-0.25  YMax=1.5~1.5  SampleTime=-1
  Sum1 : Sum  Inputs=+-|
  Terminator6 : Terminator
  Terminator7 : Terminator
  abc2albe : Subsystem
  abc2albe1 : Subsystem
  abc2dq0 PSIM : Subsystem
  Vinf_q : Outport
  Vinf_d : Outport  Port=2
  Ipac_q : Outport  Port=3
  Ipac_d : Outport  Port=4
  wires:
  Gain/1 -> Sum1/2
  I_abc/1 -> abc2albe1/1(Fabc)
  PLL/3(ro) -> PLL/2(wt), abc2dq0 PSIM/2(wt)
  DSOGI (Corrente)/1(Falbe(+)) -> PLL1/1, abc2dq0 PSIM/1(Falbe)
  DSOGI (Corrente)/2(Falbe(-)) -> Terminator7/1
  abc2albe1/1(Falbe) -> DSOGI (Corrente)/2(Falbe)
  DSOGI (Tensão)/2(Falbe(-)) -> Terminator6/1
  Vinf_abc/1 -> abc2albe/1(Fabc)
  DSOGI (Tensão)/1(Falbe(+)) -> PLL/1(Falbe)
  abc2albe/1(Falbe) -> DSOGI (Tensão)/2(Falbe)
  PLL/1(Fqd) -> Demux/1, PLL2/1
  Demux1/2 -> Ipac_d/1
  Demux/2 -> Vinf_d/1
  Demux/1 -> Vinf_q/1
  abc2dq0 PSIM/1(Fqd) -> PLL1/2, Demux1/1
  Demux1/1 -> Ipac_q/1
  PLL/2(w) -> PLL2/2
  Constant2/1 -> DSOGI (Corrente)/1(w), DSOGI (Tensão)/1(w)

== system trabalhofinal_vR2012a/PV array PI/DSOGI1/Fasor_Krause ==
  Fq : Inport
  Fd : Inport  Port=2
  Gain12 : Gain  Gain=-1
  Gain7 : Gain  Gain=1/sqrt(2)
  Real-Imag to Complex1 : RealImagToComplex
  Fasor : Outport
  wires:
  Real-Imag to Complex1/1 -> Gain7/1
  Fq/1 -> Real-Imag to Complex1/1
  Gain12/1 -> Real-Imag to Complex1/2
  Fd/1 -> Gain12/1
  Gain7/1 -> Fasor/1

== system trabalhofinal_vR2012a/PV array PI/DSOGI1/Fasor_Krause1 ==
  Fq : Inport
  Fd : Inport  Port=2
  Gain12 : Gain  Gain=-1
  Gain7 : Gain  Gain=1/sqrt(2)
  Real-Imag to Complex1 : RealImagToComplex
  Fasor : Outport
  wires:
  Gain7/1 -> Fasor/1
  Fd/1 -> Gain12/1
  Gain12/1 -> Real-Imag to Complex1/2
  Fq/1 -> Real-Imag to Complex1/1
  Real-Imag to Complex1/1 -> Gain7/1

== system trabalhofinal_vR2012a/PV array PI/PLL/abc2albe ==
  Fabc : Inport
  Gain1 : Gain  Gain=2/3  SaturateOnIntegerOverflow=on  OutDataTypeStr=Inherit: Same as input  ParamDataTypeStr=Inherit: Same as input
  Gain3 : Gain  Gain="[ 1   -1/2   -1/2; 0   sqrt(3)/2   -sqrt(3)/2 ]"  Multiplication=Matrix(K*u) (u vector)  SaturateOnIntegerOverflow=on  OutDataTypeStr=Inherit: Same as input  ParamDataTypeStr=Inherit: Same as input
  Falbe : Outport
  wires:
  Gain1/1 -> Falbe/1
  Gain3/1 -> Gain1/1
  Fabc/1 -> Gain3/1

== system trabalhofinal_vR2012a/PV array PI/PLL/abc2dq0 PSIM1 ==
  Falbe : Inport
  wt : Inport  Port=2
  Fcn1 : Fcn  Expr=u(1)*cos(u(3))+u(2)*sin(u(3))
  Fcn2 : Fcn  Expr=u(1)*sin(u(3))-u(2)*cos(u(3))
  Mux : Mux  Inputs=2
  Fq : Outport
  Fd : Outport  Port=2
  wires:
  Mux/1 -> Fcn1/1, Fcn2/1
  wt/1 -> Mux/2
  Fcn2/1 -> Fd/1
  Fcn1/1 -> Fq/1
  Falbe/1 -> Mux/1

== system trabalhofinal_vR2012a/PV array PI/abc2dq0 PSIM1/abc2albe ==
  Fabc : Inport
  Gain1 : Gain  Gain=2/3  SaturateOnIntegerOverflow=on  OutDataTypeStr=Inherit: Same as input  ParamDataTypeStr=Inherit: Same as input
  Gain3 : Gain  Gain="[ 1   -1/2   -1/2; 0   sqrt(3)/2   -sqrt(3)/2 ]"  Multiplication=Matrix(K*u) (u vector)  SaturateOnIntegerOverflow=on  OutDataTypeStr=Inherit: Same as input  ParamDataTypeStr=Inherit: Same as input
  Falbe : Outport
  wires:
  Gain1/1 -> Falbe/1
  Gain3/1 -> Gain1/1
  Fabc/1 -> Gain3/1

== system trabalhofinal_vR2012a/PV array PI/abc2dq0 PSIM1/abc2dq0 PSIM1 ==
  Falbe : Inport
  wt : Inport  Port=2
  Fcn1 : Fcn  Expr=u(1)*cos(u(3))+u(2)*sin(u(3))
  Fcn2 : Fcn  Expr=u(1)*sin(u(3))-u(2)*cos(u(3))
  Mux : Mux  Inputs=2
  Fq : Outport
  Fd : Outport  Port=2
  wires:
  Mux/1 -> Fcn1/1, Fcn2/1
  wt/1 -> Mux/2
  Fcn2/1 -> Fd/1
  Fcn1/1 -> Fq/1
  Falbe/1 -> Mux/1

== system trabalhofinal_vR2012a/PV array PI/dq02abc PSIM/abc2dq0 PSIM ==
  Fqd : Inport
  wt : Inport  Port=2
  Fcn1 : Fcn  Expr=u(1)*cos(u(3))+u(2)*sin(u(3))
  Fcn2 : Fcn  Expr=u(1)*sin(u(3))-u(2)*cos(u(3))
  Mux : Mux  Inputs=2
  Mux1 : Mux  Inputs=2
  Falbe : Outport
  wires:
  Mux1/1 -> Falbe/1
  Mux/1 -> Fcn1/1, Fcn2/1
  wt/1 -> Mux/2
  Fcn2/1 -> Mux1/2
  Fcn1/1 -> Mux1/1
  Fqd/1 -> Mux/1

== system trabalhofinal_vR2012a/PV array PI/dq02abc PSIM/albe2abc ==
  Falbe : Inport
  Gain3 : Gain  Gain="[ 1   0; -1/2  sqrt(3)/2; -1/2  -sqrt(3)/2]"  Multiplication=Matrix(K*u) (u vector)  SaturateOnIntegerOverflow=on  OutDataTypeStr=Inherit: Same as input  ParamDataTypeStr=Inherit: Same as input
  Fabc : Outport
  wires:
  Gain3/1 -> Fabc/1
  Falbe/1 -> Gain3/1

== system trabalhofinal_vR2012a/PV array Fuzzy/Compensador tensão/F1/Subsystem1 ==
  E : Inport
  Discrete Derivative1 : simulink/Discrete/Discrete Derivative  gainval=1  ICPrevScaledInput=0.0  OutMin=[]  OutMax=[]  OutDataType=fixdt(1, 16)  OutScaling=2^-10  DoSatur=off
  Gain8 : Gain  Gain=GCE
  Gain9 : Gain  Gain=GE
  Rate Transition1 : RateTransition  OutPortSampleTime=0.005
  Rate Transition2 : RateTransition  OutPortSampleTime=Ts_fuzzy
  Saturation1 : Saturate  UpperLimit=1  LowerLimit=-1
  Saturation2 : Saturate  UpperLimit=1  LowerLimit=-1
  E. : Outport
  CE : Outport  Port=2
  wires:
  Rate Transition2/1 -> CE/1
  Rate Transition1/1 -> Discrete Derivative1/1
  E/1 -> Gain9/1, Rate Transition1/1
  Saturation1/1 -> E./1
  Saturation2/1 -> Rate Transition2/1
  Gain8/1 -> Saturation2/1
  Discrete Derivative1/1 -> Gain8/1  "CE"
  Gain9/1 -> Saturation1/1

== system trabalhofinal_vR2012a/PV array Fuzzy/Compensador tensão/F2/Subsystem1 ==
  E : Inport
  Discrete Derivative1 : simulink/Discrete/Discrete Derivative  gainval=1  ICPrevScaledInput=0.0  OutMin=[]  OutMax=[]  OutDataType=fixdt(1, 16)  OutScaling=2^-10  DoSatur=off
  Gain8 : Gain  Gain=GCE
  Gain9 : Gain  Gain=GE
  Rate Transition1 : RateTransition  OutPortSampleTime=Ts_fuzzy
  Rate Transition2 : RateTransition  OutPortSampleTime=Ts_fuzzy
  Saturation1 : Saturate  UpperLimit=1  LowerLimit=-1
  Saturation2 : Saturate  UpperLimit=1  LowerLimit=-1
  E. : Outport
  CE : Outport  Port=2
  wires:
  Gain9/1 -> Saturation1/1
  Discrete Derivative1/1 -> Gain8/1  "CE"
  Gain8/1 -> Saturation2/1
  Saturation2/1 -> Rate Transition2/1
  Saturation1/1 -> E./1
  E/1 -> Rate Transition1/1, Gain9/1
  Rate Transition1/1 -> Discrete Derivative1/1
  Rate Transition2/1 -> CE/1

== system trabalhofinal_vR2012a/PV array Fuzzy/Compensador tensão/F3/Subsystem1 ==
  E : Inport
  Discrete Derivative1 : simulink/Discrete/Discrete Derivative  gainval=1  ICPrevScaledInput=0.0  OutMin=[]  OutMax=[]  OutDataType=fixdt(1, 16)  OutScaling=2^-10  DoSatur=off
  Gain8 : Gain  Gain=GCE
  Gain9 : Gain  Gain=GE
  Rate Transition1 : RateTransition  OutPortSampleTime=Ts_fuzzy
  Rate Transition2 : RateTransition  OutPortSampleTime=Ts_fuzzy
  Saturation1 : Saturate  UpperLimit=1  LowerLimit=-1
  Saturation2 : Saturate  UpperLimit=1  LowerLimit=-1
  E. : Outport
  CE : Outport  Port=2
  wires:
  Rate Transition2/1 -> CE/1
  Rate Transition1/1 -> Discrete Derivative1/1
  E/1 -> Gain9/1, Rate Transition1/1
  Saturation1/1 -> E./1
  Saturation2/1 -> Rate Transition2/1
  Gain8/1 -> Saturation2/1
  Discrete Derivative1/1 -> Gain8/1  "CE"
  Gain9/1 -> Saturation1/1

== system trabalhofinal_vR2012a/PV array Fuzzy/Compensador tensão/F4/Subsystem1 ==
  E : Inport
  Discrete Derivative1 : simulink/Discrete/Discrete Derivative  gainval=1  ICPrevScaledInput=0.0  OutMin=[]  OutMax=[]  OutDataType=fixdt(1, 16)  OutScaling=2^-10  DoSatur=off
  Gain8 : Gain  Gain=GCE
  Gain9 : Gain  Gain=GE
  Rate Transition1 : RateTransition  OutPortSampleTime=Ts_fuzzy
  Rate Transition2 : RateTransition  OutPortSampleTime=Ts_fuzzy
  Saturation1 : Saturate  UpperLimit=1  LowerLimit=-1
  Saturation2 : Saturate  UpperLimit=1  LowerLimit=-1
  E. : Outport
  CE : Outport  Port=2
  wires:
  Rate Transition2/1 -> CE/1
  Rate Transition1/1 -> Discrete Derivative1/1
  E/1 -> Gain9/1, Rate Transition1/1
  Saturation1/1 -> E./1
  Saturation2/1 -> Rate Transition2/1
  Gain8/1 -> Saturation2/1
  Discrete Derivative1/1 -> Gain8/1  "CE"
  Gain9/1 -> Saturation1/1

== system trabalhofinal_vR2012a/PV array Fuzzy/Compensador tensão/Ganhos1/Subsystem1 ==
  E : Inport
  Discrete Derivative1 : simulink/Discrete/Discrete Derivative  gainval=1  ICPrevScaledInput=0.0  OutMin=[]  OutMax=[]  OutDataType=fixdt(1, 16)  OutScaling=2^-10  DoSatur=off
  Discrete Filter : DiscreteFilter  Numerator=[2*pi*0.1e3*Ts_fuzzy 0]  Denominator=[1+2*pi*0.1e3*Ts_fuzzy -1]
  Gain8 : Gain  Gain=GCE
  Gain9 : Gain  Gain=GE
  Saturation1 : Saturate  UpperLimit=1  LowerLimit=-1
  Saturation2 : Saturate  UpperLimit=1  LowerLimit=-1
  E. : Outport
  CE : Outport  Port=2
  wires:
  E/1 -> Discrete Derivative1/1, Gain9/1
  Gain9/1 -> Saturation1/1
  Discrete Derivative1/1 -> Gain8/1  "CE"
  Gain8/1 -> Saturation2/1
  Saturation2/1 -> CE/1
  Saturation1/1 -> E./1

== system trabalhofinal_vR2012a/PV array Fuzzy/Compensador tensão/razoável/Subsystem1 ==
  E : Inport
  Discrete Derivative1 : simulink/Discrete/Discrete Derivative  gainval=1  ICPrevScaledInput=0.0  OutMin=[]  OutMax=[]  OutDataType=fixdt(1, 16)  OutScaling=2^-10  DoSatur=off
  Gain8 : Gain  Gain=GCE
  Gain9 : Gain  Gain=GE
  Saturation1 : Saturate  UpperLimit=1  LowerLimit=-1
  Saturation2 : Saturate  UpperLimit=1  LowerLimit=-1
  E. : Outport
  CE : Outport  Port=2
  wires:
  Saturation1/1 -> E./1
  Gain8/1 -> Saturation2/1
  Discrete Derivative1/1 -> Gain8/1  "CE"
  E/1 -> Discrete Derivative1/1, Gain9/1
  Saturation2/1 -> CE/1
  Gain9/1 -> Saturation1/1

== system trabalhofinal_vR2012a/PV array Fuzzy/Compensator qd-frame/FuzzyControl_q3/Subsystem1 ==
  E : Inport
  Discrete Derivative1 : simulink/Discrete/Discrete Derivative  gainval=1  ICPrevScaledInput=0.0  OutMin=[]  OutMax=[]  OutDataType=fixdt(1, 16)  OutScaling=2^-10  DoSatur=off
  Gain8 : Gain  Gain=GCE
  Gain9 : Gain  Gain=GE
  Saturation1 : Saturate  UpperLimit=1  LowerLimit=-1
  Saturation2 : Saturate  UpperLimit=1  LowerLimit=-1
  E. : Outport
  CE : Outport  Port=2
  wires:
  Gain9/1 -> Saturation1/1
  Saturation2/1 -> CE/1
  E/1 -> Gain9/1, Discrete Derivative1/1
  Discrete Derivative1/1 -> Gain8/1  "CE"
  Gain8/1 -> Saturation2/1
  Saturation1/1 -> E./1

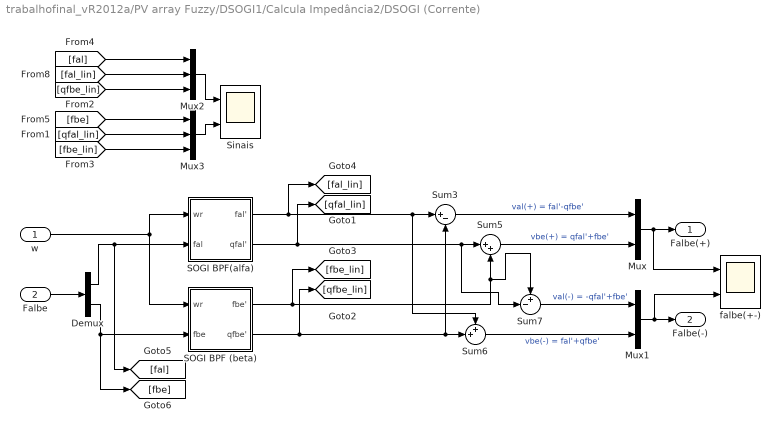
== system trabalhofinal_vR2012a/PV array Fuzzy/DSOGI1/Calcula Impedância2/DSOGI (Corrente) ==
  w : Inport
  Falbe : Inport  Port=2
  Demux : Demux  Outputs=2
  Mux : Mux  Inputs=2
  Mux1 : Mux  Inputs=2
  Mux2 : Mux  Inputs=3
  Mux3 : Mux  Inputs=3
  SOGI BPF (beta) : Subsystem
  "SOGI BPF(alfa) " : Subsystem
  Sinais : Scope  NumInputPorts=2
      settings: TimeRange=auto  MaxDataPoints=5000  SaveToWorkspace=off  SaveName=ScopeData9  YMin=-0.7~0.4  YMax=1.3~1.45  SampleTime=-1
  Sum3 : Sum  Inputs=|+-
  Sum5 : Sum  Inputs=|++
  Sum6 : Sum  Inputs=++|
  Sum7 : Sum  Inputs=+-|
  falbe(+-) : Scope  NumInputPorts=2
      settings: TimeRange=0.1  MaxDataPoints=5000  SaveToWorkspace=off  SaveName=ScopeData6  YMin=-1.5~-0.4  YMax=2~0.4  SampleTime=-1
  Falbe(+) : Outport
  Falbe(-) : Outport  Port=2
  wires:
  Mux1/1 -> falbe(+-)/2, Falbe(-)/1
  Mux/1 -> falbe(+-)/1, Falbe(+)/1
  Sum7/1 -> Mux1/1  "val(-) = -qfal'+fbe'"
  Sum6/1 -> Mux1/2  "vbe(-) = fal'+qfbe'"
  Sum5/1 -> Mux/2  "vbe(+) = qfal'+fbe'"
  Sum3/1 -> Mux/1  "val(+) = fal'-qfbe'"
  Falbe/1 -> Demux/1
  Mux2/1 -> Sinais/1
  Mux3/1 -> Sinais/2
  "SOGI BPF(alfa) "/1(fal') -> [fal_lin], Sum6/1, Sum3/1
  w/1 -> "SOGI BPF(alfa) "/1(wr), SOGI BPF (beta)/1(wr)
  Demux/1 -> [fal], "SOGI BPF(alfa) "/2(fal)
  SOGI BPF (beta)/1(fbe') -> [fbe_lin], Sum5/2, Sum7/1
  SOGI BPF (beta)/2(qfbe') -> [qfbe_lin], Sum3/2, Sum6/2
  Demux/2 -> [fbe], SOGI BPF (beta)/2(fbe)
  "SOGI BPF(alfa) "/2(qfal') -> [qfal_lin], Sum5/1, Sum7/2
  [fal_lin] -> Mux2/2
  [qfbe_lin] -> Mux2/3
  [qfal_lin] -> Mux3/2
  [fbe_lin] -> Mux3/3
  [fal] -> Mux2/1
  [fbe] -> Mux3/1

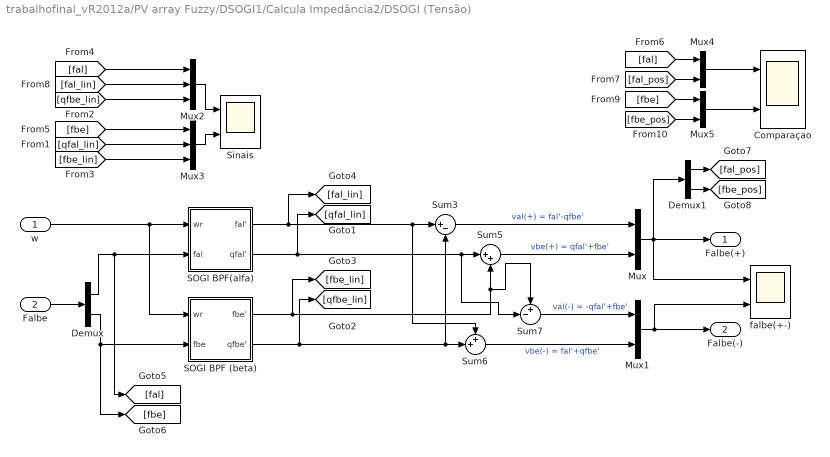
== system trabalhofinal_vR2012a/PV array Fuzzy/DSOGI1/Calcula Impedância2/DSOGI (Tensão) ==
  w : Inport
  Falbe : Inport  Port=2
  Comparaçao : Scope  NumInputPorts=2
      settings: TimeRange=auto  MaxDataPoints=5000  SaveToWorkspace=off  SaveName=ScopeData7  YMin=-0.8~-0.8  YMax=0.8~0.8  SampleTime=-1
  Demux : Demux  Outputs=2
  Demux1 : Demux  Outputs=2
  Mux{,1,4..5} (4 alike) : Mux  Inputs=2
  Mux2 : Mux  Inputs=3
  Mux3 : Mux  Inputs=3
  SOGI BPF (beta) : Subsystem
  "SOGI BPF(alfa) " : Subsystem
  Sinais : Scope  NumInputPorts=2
      settings: TimeRange=auto  MaxDataPoints=5000  SaveToWorkspace=off  SaveName=ScopeData9  YMin=-0.8~-0.8  YMax=0.8~0.8  SampleTime=-1
  Sum3 : Sum  Inputs=|+-
  Sum5 : Sum  Inputs=|++
  Sum6 : Sum  Inputs=++|
  Sum7 : Sum  Inputs=+-|
  falbe(+-) : Scope  NumInputPorts=2
      settings: TimeRange=auto  MaxDataPoints=5000  SaveToWorkspace=off  SaveName=ScopeData6  YMin=-0.8~-0.8  YMax=0.8~0.8  SampleTime=-1
  Falbe(+) : Outport
  Falbe(-) : Outport  Port=2
  wires:
  Mux1/1 -> falbe(+-)/2, Falbe(-)/1
  Mux/1 -> Demux1/1, falbe(+-)/1, Falbe(+)/1
  Sum7/1 -> Mux1/1  "val(-) = -qfal'+fbe'"
  Sum6/1 -> Mux1/2  "vbe(-) = fal'+qfbe'"
  Sum5/1 -> Mux/2  "vbe(+) = qfal'+fbe'"
  Sum3/1 -> Mux/1  "val(+) = fal'-qfbe'"
  Falbe/1 -> Demux/1
  Mux2/1 -> Sinais/1
  Mux3/1 -> Sinais/2
  "SOGI BPF(alfa) "/1(fal') -> [fal_lin], Sum6/1, Sum3/1
  w/1 -> SOGI BPF (beta)/1(wr), "SOGI BPF(alfa) "/1(wr)
  Demux/1 -> [fal], "SOGI BPF(alfa) "/2(fal)
  SOGI BPF (beta)/1(fbe') -> [fbe_lin], Sum5/2, Sum7/1
  SOGI BPF (beta)/2(qfbe') -> [qfbe_lin], Sum3/2, Sum6/2
  Demux/2 -> [fbe], SOGI BPF (beta)/2(fbe)
  "SOGI BPF(alfa) "/2(qfal') -> [qfal_lin], Sum5/1, Sum7/2
  [fal_lin] -> Mux2/2
  [qfbe_lin] -> Mux2/3
  [qfal_lin] -> Mux3/2
  [fbe_lin] -> Mux3/3
  [fal] -> Mux2/1
  [fbe] -> Mux3/1
  Mux4/1 -> Comparaçao/1
  Demux1/1 -> [fal_pos]
  Demux1/2 -> [fbe_pos]
  Mux5/1 -> Comparaçao/2
  [fal] -> Mux4/1
  [fal_pos] -> Mux4/2
  [fbe] -> Mux5/1
  [fbe_pos] -> Mux5/2

== system trabalhofinal_vR2012a/PV array Fuzzy/DSOGI1/Calcula Impedância2/PLL ==
  Falbe : Inport
  wt : Inport  Port=2
  Constant1 : Constant  Value=wB
  Constant2 : Constant  Value=wB
  Gain : Gain  Gain=-1/Vp
  Integrator : Integrator  InitialCondition=phase0_v  UpperSaturationLimit=2*pi  LowerSaturationLimit=0
  Mux : Mux  Inputs=2
  Mux1 : Mux  Inputs=2
  PID Controller : simulink/Continuous/PID Controller  Controller=PI  TimeDomain=Continuous-time  SampleTime=-1  IntegratorMethod=Forward Euler  FilterMethod=Forward Euler  Form=Parallel  UseFilter=on  ControllerParametersSource=internal  P=kp_PLL  I=ki_PLL  D=0  N=100  InitialConditionSource=internal  InitialConditionForIntegrator=0  InitialConditionForFilter=0  ExternalReset=none  LimitOutput=off  UpperSaturationLimit=inf  LowerSaturationLimit=-inf  LinearizeAsGain=on  AntiWindupMode=none  Kb=1  TrackingMode=off  Kt=1  PParamMin=[]  PParamMax=[]  IParamMin=[]  IParamMax=[]  DParamMin=[]  DParamMax=[]  NParamMin=[]  NParamMax=[]  KbParamMin=[]  KbParamMax=[]  KtParamMin=[]  KtParamMax=[]  POutMin=[]  POutMax=[]  IOutMin=[]  IOutMax=[]  DOutMin=[]  DOutMax=[]  NOutMin=[]  NOutMax=[]  KbOutMin=[]  KbOutMax=[]  KtOutMin=[]  KtOutMax=[]  IntegratorOutMin=[]  IntegratorOutMax=[]  FilterOutMin=[]  FilterOutMax=[]  SumOutMin=[]  SumOutMax=[]  SumI1OutMin=[]  SumI1OutMax=[]  SumI2OutMin=[]  SumI2OutMax=[]  SumI3OutMin=[]  SumI3OutMax=[]  SumDOutMin=[]  SumDOutMax=[]  SaturationOutMin=[]  SaturationOutMax=[]  IntegratorContinuousStateAttributes=''  IntegratorStateMustResolveToSignalObject=off  IntegratorRTWStateStorageClass=Auto  FilterContinuousStateAttributes=''  FilterStateMustResolveToSignalObject=off  FilterRTWStateStorageClass=Auto  DifferentiatorICPrevScaledInput=0  DifferentiatorOutMin=[]  DifferentiatorOutMax=[]
  PLL : Scope  NumInputPorts=4
      settings: TimeRange=auto  MaxDataPoints=5000  SaveToWorkspace=off  SaveName=ScopeData  YMin=-1.75~-0.25~7~368  YMax=1.75~1.75~15~377  SampleTime=-1
  Sum2 : Sum  Inputs=|++
  abc2dq0 PSIM : Subsystem
  Fqd : Outport
  w : Outport  Port=2
  ro : Outport  Port=3
  wires:
  wt/1 -> abc2dq0 PSIM/2(wt)
  [w] -> Mux1/1  "w"
  Integrator/1 -> [ro], ro/1
  abc2dq0 PSIM/2(Fd) -> Gain/1, Mux/2
  [Falbe] -> PLL/1  "Falbe"
  Falbe/1 -> [Falbe], abc2dq0 PSIM/1(Falbe)
  [ro] -> PLL/3  "ro"
  [Fqd] -> PLL/2  "Fqd"
  Constant2/1 -> Sum2/2
  Mux/1 -> Fqd/1, [Fqd]
  abc2dq0 PSIM/1(Fq) -> Mux/1
  Sum2/1 -> Integrator/1, w/1, [w]
  Gain/1 -> PID Controller/1
  Mux1/1 -> PLL/4
  Constant1/1 -> Mux1/2
  PID Controller/1 -> Sum2/1

== system trabalhofinal_vR2012a/PV array Fuzzy/DSOGI1/Calcula Impedância2/abc2albe ==
  Fabc : Inport
  Gain1 : Gain  Gain=2/3  SaturateOnIntegerOverflow=on  OutDataTypeStr=Inherit: Same as input  ParamDataTypeStr=Inherit: Same as input
  Gain3 : Gain  Gain="[ 1   -1/2   -1/2; 0   sqrt(3)/2   -sqrt(3)/2 ]"  Multiplication=Matrix(K*u) (u vector)  SaturateOnIntegerOverflow=on  OutDataTypeStr=Inherit: Same as input  ParamDataTypeStr=Inherit: Same as input
  Falbe : Outport
  wires:
  Gain1/1 -> Falbe/1
  Gain3/1 -> Gain1/1
  Fabc/1 -> Gain3/1

== system trabalhofinal_vR2012a/PV array Fuzzy/DSOGI1/Calcula Impedância2/abc2albe1 ==
  Fabc : Inport
  Gain1 : Gain  Gain=2/3  SaturateOnIntegerOverflow=on  OutDataTypeStr=Inherit: Same as input  ParamDataTypeStr=Inherit: Same as input
  Gain3 : Gain  Gain="[ 1   -1/2   -1/2; 0   sqrt(3)/2   -sqrt(3)/2 ]"  Multiplication=Matrix(K*u) (u vector)  SaturateOnIntegerOverflow=on  OutDataTypeStr=Inherit: Same as input  ParamDataTypeStr=Inherit: Same as input
  Falbe : Outport
  wires:
  Fabc/1 -> Gain3/1
  Gain3/1 -> Gain1/1
  Gain1/1 -> Falbe/1

== system trabalhofinal_vR2012a/PV array Fuzzy/DSOGI1/Calcula Impedância2/abc2dq0 PSIM ==
  Falbe : Inport
  wt : Inport  Port=2
  Fcn1 : Fcn  Expr=u(1)*cos(u(3))+u(2)*sin(u(3))
  Fcn2 : Fcn  Expr=u(1)*sin(u(3))-u(2)*cos(u(3))
  Mux : Mux  Inputs=2
  Mux1 : Mux  Inputs=2
  Fqd : Outport
  wires:
  Mux1/1 -> Fqd/1
  Mux/1 -> Fcn1/1, Fcn2/1
  wt/1 -> Mux/2
  Fcn2/1 -> Mux1/2
  Fcn1/1 -> Mux1/1
  Falbe/1 -> Mux/1

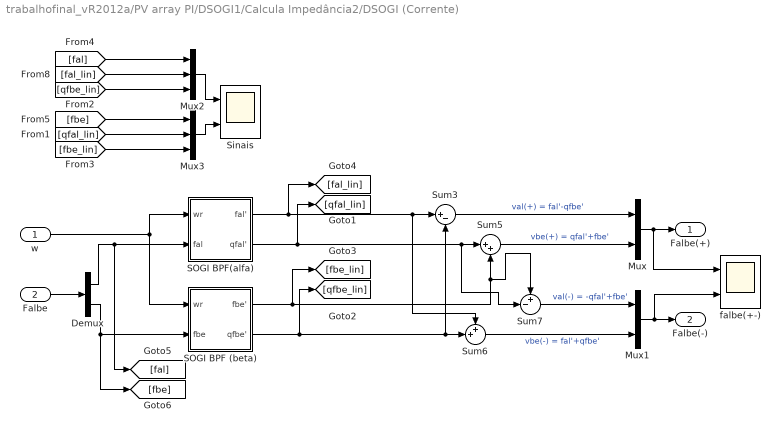
== system trabalhofinal_vR2012a/PV array PI/DSOGI1/Calcula Impedância2/DSOGI (Corrente) ==
  w : Inport
  Falbe : Inport  Port=2
  Demux : Demux  Outputs=2
  Mux : Mux  Inputs=2
  Mux1 : Mux  Inputs=2
  Mux2 : Mux  Inputs=3
  Mux3 : Mux  Inputs=3
  SOGI BPF (beta) : Subsystem
  "SOGI BPF(alfa) " : Subsystem
  Sinais : Scope  NumInputPorts=2
      settings: TimeRange=auto  MaxDataPoints=5000  SaveToWorkspace=off  SaveName=ScopeData9  YMin=-0.7~0.4  YMax=1.3~1.45  SampleTime=-1
  Sum3 : Sum  Inputs=|+-
  Sum5 : Sum  Inputs=|++
  Sum6 : Sum  Inputs=++|
  Sum7 : Sum  Inputs=+-|
  falbe(+-) : Scope  NumInputPorts=2
      settings: TimeRange=0.1  MaxDataPoints=5000  SaveToWorkspace=off  SaveName=ScopeData6  YMin=-1.5~-0.4  YMax=2~0.4  SampleTime=-1
  Falbe(+) : Outport
  Falbe(-) : Outport  Port=2
  wires:
  Mux1/1 -> falbe(+-)/2, Falbe(-)/1
  Mux/1 -> falbe(+-)/1, Falbe(+)/1
  Sum7/1 -> Mux1/1  "val(-) = -qfal'+fbe'"
  Sum6/1 -> Mux1/2  "vbe(-) = fal'+qfbe'"
  Sum5/1 -> Mux/2  "vbe(+) = qfal'+fbe'"
  Sum3/1 -> Mux/1  "val(+) = fal'-qfbe'"
  Falbe/1 -> Demux/1
  Mux2/1 -> Sinais/1
  Mux3/1 -> Sinais/2
  "SOGI BPF(alfa) "/1(fal') -> [fal_lin], Sum6/1, Sum3/1
  w/1 -> "SOGI BPF(alfa) "/1(wr), SOGI BPF (beta)/1(wr)
  Demux/1 -> [fal], "SOGI BPF(alfa) "/2(fal)
  SOGI BPF (beta)/1(fbe') -> [fbe_lin], Sum5/2, Sum7/1
  SOGI BPF (beta)/2(qfbe') -> [qfbe_lin], Sum3/2, Sum6/2
  Demux/2 -> [fbe], SOGI BPF (beta)/2(fbe)
  "SOGI BPF(alfa) "/2(qfal') -> [qfal_lin], Sum5/1, Sum7/2
  [fal_lin] -> Mux2/2
  [qfbe_lin] -> Mux2/3
  [qfal_lin] -> Mux3/2
  [fbe_lin] -> Mux3/3
  [fal] -> Mux2/1
  [fbe] -> Mux3/1

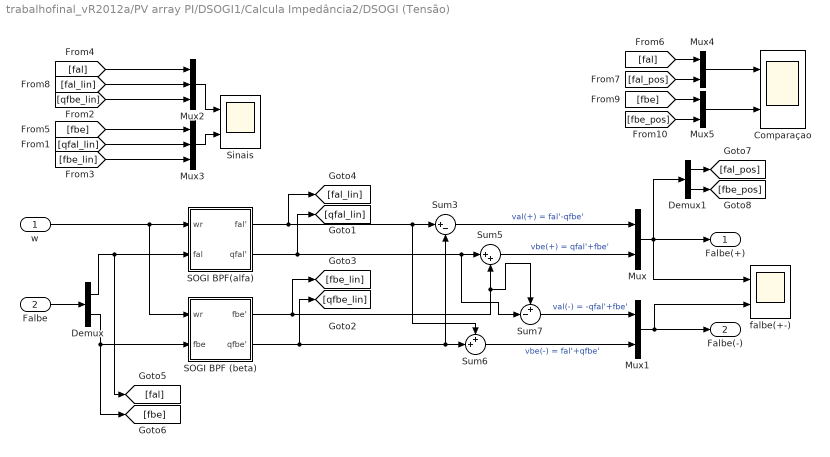
== system trabalhofinal_vR2012a/PV array PI/DSOGI1/Calcula Impedância2/DSOGI (Tensão) ==
  w : Inport
  Falbe : Inport  Port=2
  Comparaçao : Scope  NumInputPorts=2
      settings: TimeRange=auto  MaxDataPoints=5000  SaveToWorkspace=off  SaveName=ScopeData7  YMin=-0.8~-0.8  YMax=0.8~0.8  SampleTime=-1
  Demux : Demux  Outputs=2
  Demux1 : Demux  Outputs=2
  Mux{,1,4..5} (4 alike) : Mux  Inputs=2
  Mux2 : Mux  Inputs=3
  Mux3 : Mux  Inputs=3
  SOGI BPF (beta) : Subsystem
  "SOGI BPF(alfa) " : Subsystem
  Sinais : Scope  NumInputPorts=2
      settings: TimeRange=auto  MaxDataPoints=5000  SaveToWorkspace=off  SaveName=ScopeData9  YMin=-0.8~-0.8  YMax=0.8~0.8  SampleTime=-1
  Sum3 : Sum  Inputs=|+-
  Sum5 : Sum  Inputs=|++
  Sum6 : Sum  Inputs=++|
  Sum7 : Sum  Inputs=+-|
  falbe(+-) : Scope  NumInputPorts=2
      settings: TimeRange=auto  MaxDataPoints=5000  SaveToWorkspace=off  SaveName=ScopeData6  YMin=-0.8~-0.8  YMax=0.8~0.8  SampleTime=-1
  Falbe(+) : Outport
  Falbe(-) : Outport  Port=2
  wires:
  Mux1/1 -> falbe(+-)/2, Falbe(-)/1
  Mux/1 -> Demux1/1, falbe(+-)/1, Falbe(+)/1
  Sum7/1 -> Mux1/1  "val(-) = -qfal'+fbe'"
  Sum6/1 -> Mux1/2  "vbe(-) = fal'+qfbe'"
  Sum5/1 -> Mux/2  "vbe(+) = qfal'+fbe'"
  Sum3/1 -> Mux/1  "val(+) = fal'-qfbe'"
  Falbe/1 -> Demux/1
  Mux2/1 -> Sinais/1
  Mux3/1 -> Sinais/2
  "SOGI BPF(alfa) "/1(fal') -> [fal_lin], Sum6/1, Sum3/1
  w/1 -> SOGI BPF (beta)/1(wr), "SOGI BPF(alfa) "/1(wr)
  Demux/1 -> [fal], "SOGI BPF(alfa) "/2(fal)
  SOGI BPF (beta)/1(fbe') -> [fbe_lin], Sum5/2, Sum7/1
  SOGI BPF (beta)/2(qfbe') -> [qfbe_lin], Sum3/2, Sum6/2
  Demux/2 -> [fbe], SOGI BPF (beta)/2(fbe)
  "SOGI BPF(alfa) "/2(qfal') -> [qfal_lin], Sum5/1, Sum7/2
  [fal_lin] -> Mux2/2
  [qfbe_lin] -> Mux2/3
  [qfal_lin] -> Mux3/2
  [fbe_lin] -> Mux3/3
  [fal] -> Mux2/1
  [fbe] -> Mux3/1
  Mux4/1 -> Comparaçao/1
  Demux1/1 -> [fal_pos]
  Demux1/2 -> [fbe_pos]
  Mux5/1 -> Comparaçao/2
  [fal] -> Mux4/1
  [fal_pos] -> Mux4/2
  [fbe] -> Mux5/1
  [fbe_pos] -> Mux5/2
